simulink model "question2_model"  (R2018a)
settings: Solver=FixedStepAuto  StartTime=0.0  StopTime=100  RelTol=1e-5
settings Model: Creator=Emre Deniz  LastModifiedBy=Emre Deniz

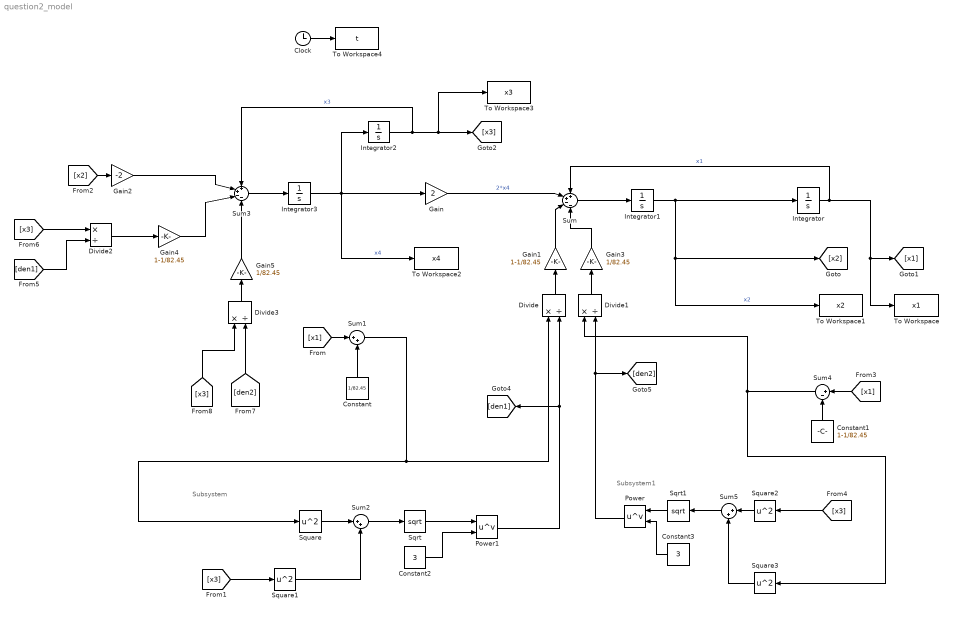
== system question2_model ==
  note: Subsystem1
  note: Subsystem
  Clock : Clock
  Constant : Constant  Value=1/82.45
  Constant1 : Constant  Value=1-1/82.45
  Constant2 : Constant  Value=3
  Constant3 : Constant  Value=3
  Divide{,1..3} (4 alike) : Product  Inputs=*/
  Gain : Gain  Gain=2
  Gain1 : Gain  Gain=1-1/82.45
  Gain2 : Gain  Gain=-2
  Gain3 : Gain  Gain=1/82.45
  Gain4 : Gain  Gain=1-1/82.45
  Gain5 : Gain  Gain=1/82.45
  Integrator : Integrator  InitialCondition=1.2
  Integrator1 : Integrator
  Integrator2 : Integrator
  Integrator3 : Integrator  InitialCondition=-1.0494
  Power : Math  Operator=pow  SaturateOnIntegerOverflow=on
  Power1 : Math  Operator=pow  SaturateOnIntegerOverflow=on
  Sqrt : Sqrt  SaturateOnIntegerOverflow=on
  Sqrt1 : Sqrt  SaturateOnIntegerOverflow=on
  Square{,1..3} (4 alike) : Math  Operator=square  SaturateOnIntegerOverflow=on
  Sum : Sum  Inputs=++--
  Sum1 : Sum  Inputs=|++
  Sum2 : Sum  Inputs=|++
  Sum3 : Sum  Inputs=++--
  Sum4 : Sum  Inputs=|+-
  Sum5 : Sum  Inputs=|++
  To Workspace : ToWorkspace  VariableName=x1  SampleTime=-1
  To Workspace1 : ToWorkspace  VariableName=x2  SampleTime=-1
  To Workspace2 : ToWorkspace  VariableName=x4  SampleTime=-1
  To Workspace3 : ToWorkspace  VariableName=x3  SampleTime=-1
  To Workspace4 : ToWorkspace  VariableName=t  SampleTime=-1
  wires:
  Integrator/1 -> To Workspace/1, [x1], Sum/1  "x1"
  Integrator1/1 -> To Workspace1/1, [x2], Integrator/1  "x2"
  Gain/1 -> Sum/2  "2*x4"
  Integrator3/1 -> Integrator2/1, Gain/1, To Workspace2/1  "x4"
  Gain1/1 -> Sum/3
  Sum/1 -> Integrator1/1
  [x1] -> Sum1/1
  Constant/1 -> Sum1/2
  Divide/1 -> Gain1/1
  Integrator2/1 -> Sum3/1, [x3], To Workspace3/1  "x3"
  Sum3/1 -> Integrator3/1
  Gain2/1 -> Sum3/2
  [x2] -> Gain2/1
  [x1] -> Sum4/1
  Constant1/1 -> Sum4/2
  Gain3/1 -> Sum/4
  Divide1/1 -> Gain3/1
  Gain4/1 -> Sum3/3
  Gain5/1 -> Sum3/4
  Divide3/1 -> Gain5/1
  Divide2/1 -> Gain4/1
  [den1] -> Divide2/2
  [x3] -> Divide2/1
  [den2] -> Divide3/2
  [x3] -> Divide3/1
  Clock/1 -> To Workspace4/1
  Power1/1 -> Divide/2, [den1]
  Power/1 -> Divide1/2, [den2]
  Sum1/1 -> Square/1, Divide/1
  Sqrt/1 -> Power1/1
  Sum2/1 -> Sqrt/1
  Square1/1 -> Sum2/2
  [x3] -> Square1/1
  Square/1 -> Sum2/1
  Constant2/1 -> Power1/2
  Sum4/1 -> Square3/1, Divide1/1
  Constant3/1 -> Power/2
  [x3] -> Square2/1
  Sqrt1/1 -> Power/1
  Sum5/1 -> Sqrt1/1
  Square2/1 -> Sum5/1
  Square3/1 -> Sum5/2
